simulink model "darshan_soqpsk_try"  (R2022b)
settings: Solver=VariableStepAuto  StartTime=0.0  StopTime=10.0  RelTol=1e-3
libraries: commrandsrc3 x1
settings Model: Creator=Devika  LastModifiedBy=darsh
settings SolverCC: AlgebraicLoopSolver=TrustRegion
settings DataIOCC: ReturnWorkspaceOutputs=off
settings DebuggingCC: UnconnectedInputMsg=warning  UnconnectedOutputMsg=warning  UnconnectedLineMsg=warning  SFMachineParentedDataDiag=warning  ArithmeticOperatorsInVariantConditions=warning
settings ModelReferenceCC: EnableRefExpFcnMdlSchedulingChecks=on
settings SFSimCC: SimUseLocalCustomCode=off  CustomCodeUndefinedFunction=UseInterfaceOnly
settings RTWCC: RTWUseLocalCustomCode=off

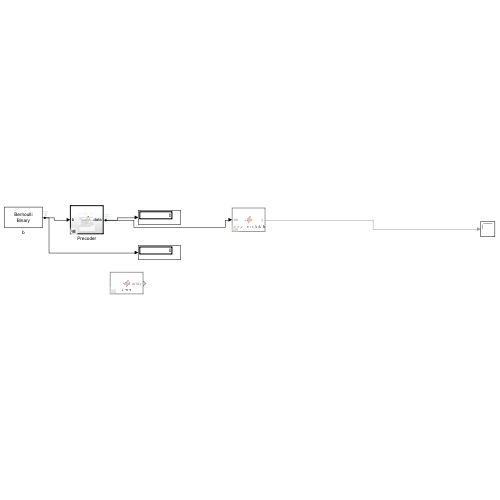
[thumbnail: Simulink's stored preview of the top-level diagram]
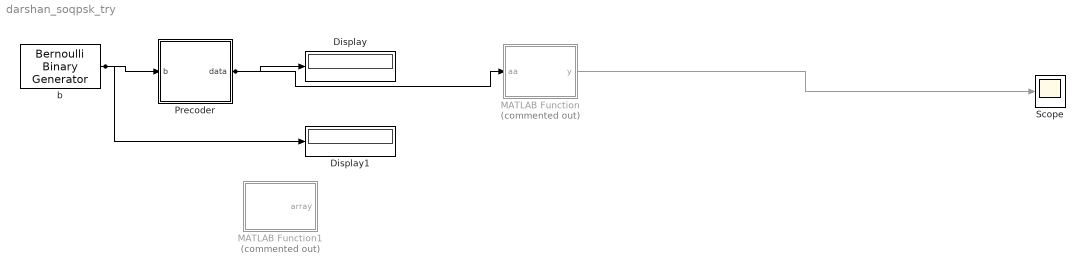
== system darshan_soqpsk_try ==
  Display : Display
  Display1 : Display
  MATLAB Function : MATLAB Function  Commented=on  TreatAsAtomicUnit=on
  MATLAB Function1 : MATLAB Function  Commented=on  TreatAsAtomicUnit=on
  Precoder : Subsystem  TreatAsAtomicUnit=on  Variant=on  VariantControlMode=label  VariantControl=Choice  LabelModeActiveChoice=(default)
  Scope : Scope
  b : commrandsrc3/Bernoulli Binary Generator  ProbabilityOfZero=0.5  SeedSource=Auto  Seed=0  SampleTime=1e-2  SamplesPerFrame=1  OutputDataType=double  SimulateUsing=Interpreted execution
  wires:
  b/1 -> Display1/1, Precoder/1(b)
  MATLAB Function/1(y) -> Scope/1
  Precoder/1(data) -> MATLAB Function/1(aa), Display/1

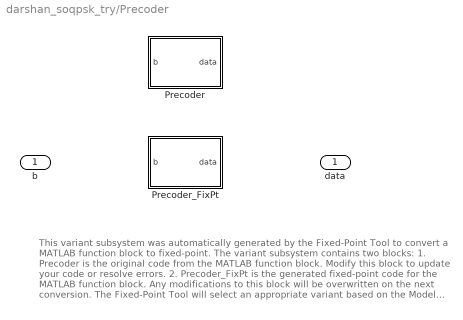
== system darshan_soqpsk_try/Precoder ==
  note: This variant subsystem was automatically generated by the Fixed-Point Tool to convert a MATLAB function block to fixed-point.
      |
      | The variant subsystem contains two blocks:
      | 1. Precoder is the original code from the MATLAB function block. Modify this block to update your code or resolve errors.
      |
      | 2. Precoder_FixPt is the generated fixed-point code for the MATLAB function block. Any modifications to this block will be overwritten on the next conversion.
      |
      | The Fixed-Point Tool will select an appropriate variant based on the Model Settings. Learn more. .
  b : Inport
  Precoder : MATLAB Function  TreatAsAtomicUnit=on  VariantControl=false()
  Precoder_FixPt : MATLAB Function  TreatAsAtomicUnit=on  VariantControl=(default)
  data : Outport

== matlab function darshan_soqpsk_try/MATLAB Function ==
  data: aa input size=1; y output
function y = soqpsk_modulator(aa)
%#codegen

Nb=10;
freq = SOQPSK_frequency_pulse_internal(Nb);
temp = zeros(1,Nb*(length(aa)-1)+1);
temp(1:Nb:end) = aa;
dphi = pi*conv(temp,freq);                          %2*pi*h=pi (h=1/2)
phi = filter([0 1],[1 -1],dphi) + 3*pi/2 - pi/4;
y=exp(1i*phi);
                                                            % An additional -pi/4 phase shift is added to 
                                                            % generate nice looking I/Q eye diagrams


function f = SOQPSK_frequency_pulse_internal(N)
%#codegen
rho = 0.7;                                                 %parameters according to SOQPSK-B
B = 1.25;
T1 = 1.5;
T2 = 0.5;

n1 = 0:2*N*T1-1;                                           %0<mod(t/2Ts)<T1
n2 = 2*N*T1:2*N*(T1+T2);                                   %T1<mod(t/2Ts)<T1+T2
nall = [n1 n2]; 
part1 = cos(pi*rho*B*nall/(2*N)) ./ (1-4*(rho*B*nall/(2*N)).^2);
part2 = sinc(B*nall/(2*N));
w = [ones(size(n1)) 0.5*(1+cos(pi/T2*(n2/(2*N)-T1)))];%plot(w);

temp = part1 .* part2 .* w; 
%plot(temp);                   %g(t)=n(t)*w(t)
f = [temp(end:-1:2) temp]; 
f = f*0.5/sum(f);

== matlab function darshan_soqpsk_try/MATLAB Function1 ==
  data: array output
function array =  cpm
%#codegen
array
end

== matlab function darshan_soqpsk_try/Precoder/Precoder_FixPt ==
  settings: fimath=fimath('RoundingMethod', 'Floor', 'OverflowAction', 'Wrap', 'ProductMode', 'FullPrecision', 'MaxProductWordLength', 128, 'SumMode', 'FullPrecision', 'MaxSumWordLength', 128)
  data: b input size=1; data output size=1
%auto-generated
function data = precoder_fixpt(b)
%#codegen

fm = get_fimath();
b = fi(b, 0, 16, 15, fm);

a=fi(fi_signed(fi(2, 0, 2, 0, fm)*b)-fi(1, 0, 1, 0, fm), 1, 16, 14, fm);
persistent n;
if isempty(n)
        n = fi(0, 0, 16, 6, fm);
end
n(:)=n+fi(1, 0, 1, 0, fm);
persistent d;
if isempty(d)
        d = fi(0, 1, 16, 4, fm);
end
persistent d2;
if isempty(d2)
        d2 = fi(0, 1, 16, 4, fm);
end
switch(n)
    case fi(1, 0, 1, 0, fm)
        data = fi(fi(0*5*(-1), 0, 1, 0, fm)*(a(1)+fi(1, 0, 1, 0, fm)), 1, 16, 4, fm);
    case fi(2, 0, 2, 0, fm)
        data = fi(fi(0.5, 0, 16, 16, fm)*d*(a+fi(1, 0, 1, 0, fm)), 1, 16, 4, fm);
    otherwise
        data = fi(fi(0.5, 0, 16, 16, fm)*d*(a-d2), 1, 16, 4, fm);       
end
d2(:)=d;
d(:)=data;
end



function y = fi_signed(a)
    coder.inline( 'always' );
    if isfi( a ) && ~(issigned( a ))
        nt = numerictype( a );
        new_nt = numerictype( 1, nt.WordLength + 1, nt.FractionLength );
        y = fi( a, new_nt, fimath( a ) );
    else
        y = a;
    end
end

function fm = get_fimath()
	fm = fimath('RoundingMethod', 'Floor',...
	     'OverflowAction', 'Wrap',...
	     'ProductMode','FullPrecision',...
	     'MaxProductWordLength', 128,...
	     'SumMode','FullPrecision',...
	     'MaxSumWordLength', 128);
end

== matlab function darshan_soqpsk_try/Precoder/Precoder ==
  data: b input size=1; data output size=1
function data = precoder(b)
%#codegen

a=2*b-1;
persistent n;
if isempty(n)
        n = 0;
end
n=n+1;
persistent d;
if isempty(d)
        d = 0;
end
persistent d2;
if isempty(d2)
        d2 = 0;
end
switch(n)
    case 1
        data = 0*5*(-1)*(a(1)+1);
    case 2
        data = 0.5*d*(a+1);
    otherwise
        data = 0.5*d*(a-d2);       
end
d2=d;
d=data;
end
